simulink model "Discrete_FIR_Filter"  (R2023b)
settings: Solver=VariableStepAuto  StartTime=0.0  StopTime=2  RelTol=1e-3
values from neighbouring files (symbols this model uses):
  h1 = load('h1.txt')    [Exp1_FIR_Filter.m]
  h2 = load('h2.txt')    [Exp1_FIR_Filter.m]
settings Model: Creator=carlo  LastModifiedBy=carlo

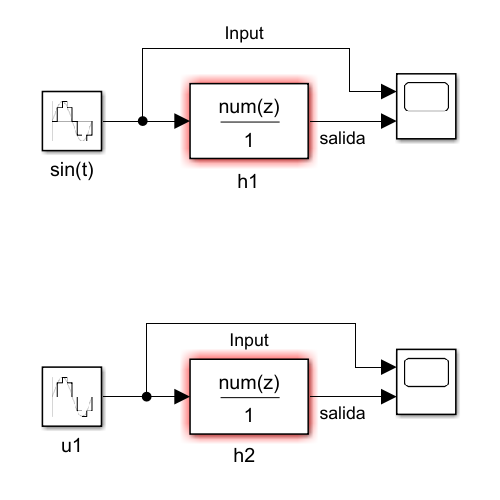
[thumbnail: Simulink's stored preview of the top-level diagram]
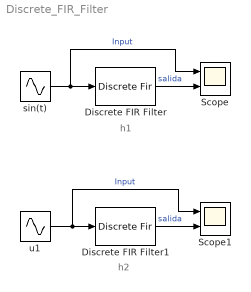
== system Discrete_FIR_Filter ==
  note: h2
  note: h1
  Discrete FIR Filter : DiscreteFir  Coefficients=h1  SampleTime=1/250
  Discrete FIR Filter1 : DiscreteFir  Coefficients=h2  SampleTime=1/250
  Scope : Scope  NumInputPorts=2
  Scope1 : Scope  NumInputPorts=2
  sin(t) : Sin  Frequency=80*2*pi  SampleTime=1/250
  u1 : Sin  Frequency=9*2*pi  SampleTime=1/250
  wires:
  sin(t)/1 -> Scope/1, Discrete FIR Filter/1  "Input"
  u1/1 -> Scope1/1, Discrete FIR Filter1/1  "Input"
  Discrete FIR Filter/1 -> Scope/2  "salida"
  Discrete FIR Filter1/1 -> Scope1/2  "salida"
